simulink model "damper"  (R2019a)
settings: Solver=VariableStepAuto  StartTime=0.0  StopTime=10.0  MaxStep=1e-3  RelTol=1e-3
settings Model: Creator=Frieder Uerlings  LastModifiedBy=Frieder Uerlings

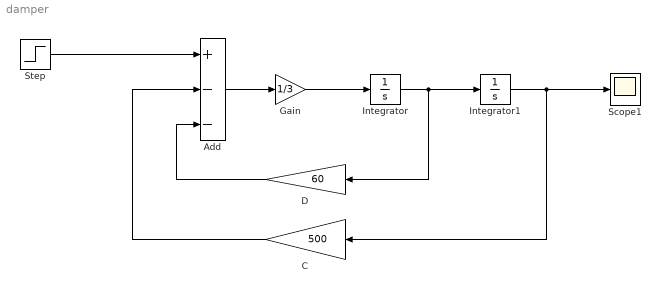
== system damper ==
  Add : Sum  Inputs=+--
  C : Gain  Gain=500
  "D " : Gain  Gain=60
  Gain : Gain  Gain=1/3
  Integrator : Integrator
  Integrator1 : Integrator
  Scope1 : Scope
  Step : Step  After=500  SampleTime=0
  wires:
  Add/1 -> Gain/1
  Gain/1 -> Integrator/1
  Integrator/1 -> "D "/1, Integrator1/1
  "D "/1 -> Add/3
  C/1 -> Add/2
  Step/1 -> Add/1
  Integrator1/1 -> Scope1/1, C/1
